simulink model "station1_task"  (Simulink 3.00)
libraries: mathlib x2, execlib x2, analoglib x1, logiclib x1, paramlib x1, speclib x1
settings Model: rev.=3173,  Date=2013-05-31

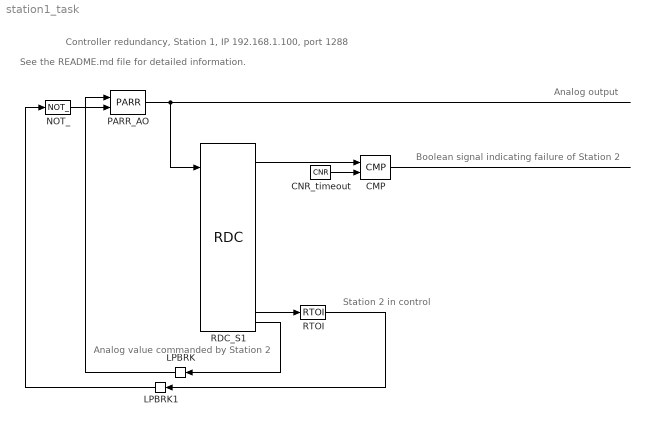
== system station1_task ==
  note: Controller redundancy, Station 1, IP 192.168.1.100, port 1288
  note: See the README.md file for detailed information.
  note: Boolean signal indicating failure of Station 2
  note: Station 2 in control
  note: Analog output
  note: Analog value commanded by Station 2
  CMP : analoglib/CMP  hys=0
  CNR_timeout : mathlib/CNR  ycn=5
  LPBRK : execlib/LPBRK  Orientation=left
  LPBRK1 : execlib/LPBRK  Orientation=left
  NOT_ : logiclib/NOT_
  PARR_AO : paramlib/PARR  par=3.7  SATF=off  hilim=1  lolim=-1
  RDC_S1 : speclib/RDC  target=192.168.1.200  rport=1288  lport=1288  id=1  period=0.5
  RTOI : mathlib/RTOI
  wires:
  CMP/1 -> ?
  CNR_timeout/1 -> CMP/2
  LPBRK/1 -> PARR_AO/1
  LPBRK1/1 -> NOT_/1
  NOT_/1 -> PARR_AO/2
  PARR_AO/1 -> RDC_S1/2
  RDC_S1/2 -> CMP/1
  RDC_S1/17 -> RTOI/1
  RDC_S1/18 -> LPBRK/1
  RTOI/1 -> LPBRK1/1
